simulink model "cicSimuBlocksSine"  (R2017a)
settings: Solver=FixedStepAuto  StartTime=0.0  StopTime=200  FixedStep=1  RelTol=1e-3
libraries: dspsrcs4 x1
settings Model: Creator=of-1  LastModifiedBy=of-1
settings DataIOCC: SaveFormat=Array  TimeSaveName=t_out  OutputSaveName=y_out

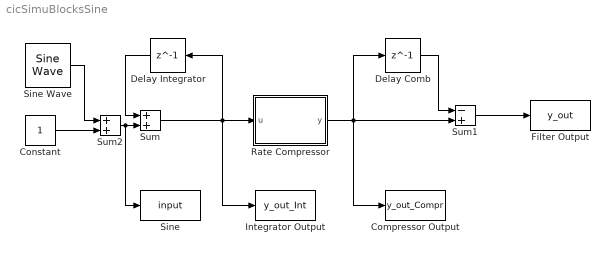
== system cicSimuBlocksSine ==
  Compressor Output : ToWorkspace  VariableName=y_out_Compr  SampleTime=2
      settings: Save2DSignal=2-D array (concatenate along first dimension)
  Constant : Constant  OutDataTypeStr=fixdt(1,3,0)  SampleTime=1
  Delay Comb : Delay  DelayLength=1  InitialCondition=0  SampleTime=2
  Delay Integrator : Delay  DelayLength=1  InitialCondition=0  SampleTime=1
  Filter Output : ToWorkspace  VariableName=y_out  SampleTime=2
      settings: Save2DSignal=2-D array (concatenate along first dimension)
  Integrator Output : ToWorkspace  VariableName=y_out_Int  SampleTime=1
      settings: Save2DSignal=2-D array (concatenate along first dimension)
  Rate Compressor : MATLAB Function  TreatAsAtomicUnit=on
  Sine : ToWorkspace  VariableName=input  SampleTime=1
      settings: Save2DSignal=2-D array (concatenate along first dimension)
  Sine Wave : dspsrcs4/Sine Wave  Amplitude=16  Frequency=1/20  Phase=0  SampleMode=Discrete  OutComplex=Real  CompMethod=Table lookup  TableSize=Speed  SampleTime=1  SamplesPerFrame=1  ResetState=Restart at time zero  OutputFrames=off  dataType=Fixed-point  wordLen=6  udDataType=sfix(16)  fracBitsMode=User-defined  numFracBits=0  OutDataTypeStr=fixdt(1,6,0)  LastOutDataTypeStr=fixdt(1,6,0)
  Sum : Sum  AccumDataTypeStr=fixdt(1,6,0)  OutDataTypeStr=fixdt(1,6,0)
  Sum1 : Sum  Inputs=-+  AccumDataTypeStr=fixdt(1,6,0)  OutDataTypeStr=fixdt(1,6,0)
  Sum2 : Sum  AccumDataTypeStr=fixdt(1,6,0)  OutDataTypeStr=fixdt(1,6,0)
  wires:
  Delay Integrator/1 -> Sum/1
  Sum/1 -> Integrator Output/1, Rate Compressor/1(u), Delay Integrator/1
  Delay Comb/1 -> Sum1/1
  Sum1/1 -> Filter Output/1
  Rate Compressor/1(y) -> Compressor Output/1, Delay Comb/1, Sum1/2
  Constant/1 -> Sum2/2
  Sum2/1 -> Sine/1, Sum/2
  Sine Wave/1 -> Sum2/1

== matlab function cicSimuBlocksSine/Rate Compressor ==
  data: u input; y output
function y = fcn(u)

y = u(1:2:length(u));

end
